simulink model "crazy_model_LQR"  (R2014b)
settings: Solver=ode4  StartTime=0.0  StopTime=1  FixedStep=0.01  RelTol=1e-3
values from neighbouring files (symbols this model uses):
  Engine_back = 1.3    [main.m]
  Engine_front = 1.3    [main.m]
  Engine_left = 1.3    [main.m]
  Engine_right = 1.3    [main.m]
  Klqr = [-0.0000   -0.5502   -0.0000   -0.0000   -0.0516   -0.0000    0.0000   -0.8559    0.6891    0.0000   -0.2911    0.2725 ... (first row only)    [C_code_Klqr.m]    (also in main.m = lqr(A,B,Qx,Qu))
  Kv = 14000*[1 0 0 0 ... (first row only)    [control_PWM.m]    (also in linearize_pwm.m = 14000; linearize_voltage.m = 14000; main.m)
settings Model: Creator=Abhiram  LastModifiedBy=Abhiram

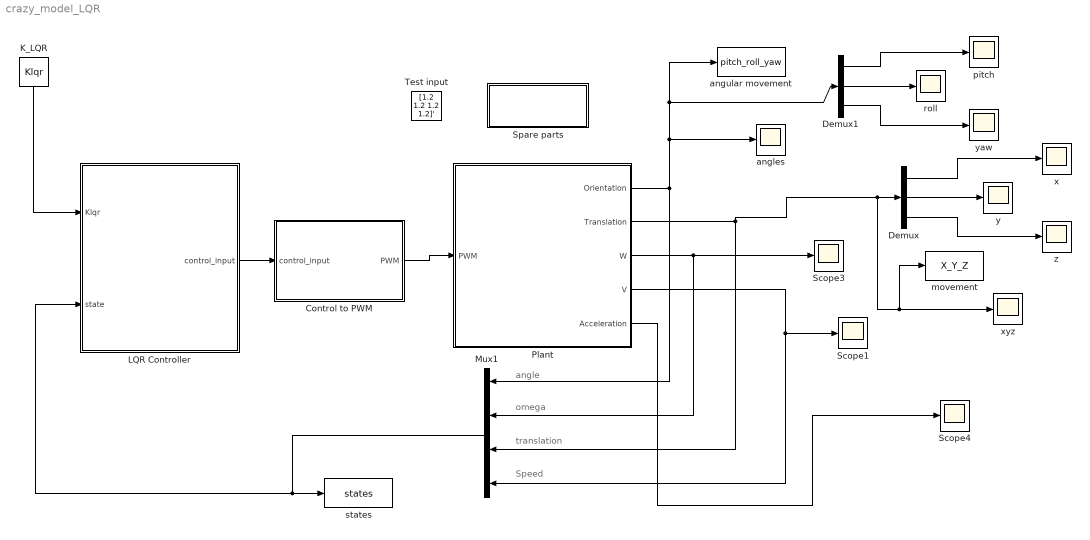
== system crazy_model_LQR ==
  note: Speed
  note: translation
  note: omega
  note: angle
  Control to PWM : MATLAB Function  TreatAsAtomicUnit=on
  Demux : Demux  Outputs=3
  Demux1 : Demux  Outputs=3
  K_LQR : Constant  Value=Klqr
  LQR Controller : MATLAB Function  TreatAsAtomicUnit=on
  Mux1 : Mux
  Plant : Subsystem
  Scope1 : Scope
  Scope3 : Scope
      settings: SaveName=ScopeData3
  Scope4 : Scope
      settings: SaveName=ScopeData4
  Spare parts : Subsystem
  Test input : Constant  Value=[1.2 1.2 1.2 1.2]'
  angles : Scope
      settings: SaveName=ScopeData10
  angular movement : ToWorkspace  VariableName=pitch_roll_yaw  SaveFormat=Structure With Time  SampleTime=-1
  movement : ToWorkspace  VariableName=X_Y_Z  SaveFormat=Structure With Time  SampleTime=-1
  pitch : Scope
  roll : Scope
      settings: TimeRange=10  YMin=0  YMax=25  SaveName=ScopeData7
  states : ToWorkspace  VariableName=states  SaveFormat=Structure With Time  SampleTime=-1
  x : Scope
      settings: SaveName=ScopeData2
  xyz : Scope
      settings: TimeRange=10  YMin=-20  YMax=120  SaveName=ScopeData9
  y : Scope
      settings: SaveName=ScopeData5
  yaw : Scope
      settings: SaveName=ScopeData8
  z : Scope
      settings: SaveName=ScopeData6
  wires:
  Plant/1(Orientation) -> angular movement/1, Demux1/1, angles/1, Mux1/1
  Plant/3(W) -> Mux1/2, Scope3/1
  Plant/4(V) -> Mux1/4, Scope1/1
  Plant/5(Acceleration) -> Scope4/1
  Plant/2(Translation) -> Demux/1, movement/1, xyz/1, Mux1/3
  Demux/1 -> x/1
  Demux/2 -> y/1
  Demux/3 -> z/1
  Demux1/1 -> pitch/1
  Demux1/2 -> roll/1
  Demux1/3 -> yaw/1
  Mux1/1 -> states/1, LQR Controller/2(state)
  Control to PWM/1(PWM) -> Plant/1(PWM)
  LQR Controller/1(control_input) -> Control to PWM/1(control_input)
  K_LQR/1 -> LQR Controller/1(Klqr)

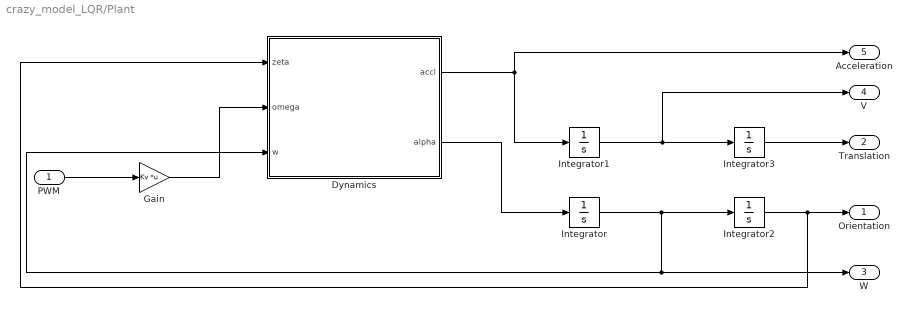
== system crazy_model_LQR/Plant ==
  PWM : Inport
  Dynamics : MATLAB Function  TreatAsAtomicUnit=on
  Gain : Gain  Gain=Kv  Multiplication=Matrix(K*u)
  Integrator{,1..3} (4 alike) : Integrator  InitialCondition=[0 0 0]'
  Orientation : Outport
  Translation : Outport  Port=2
  W : Outport  Port=3
  V : Outport  Port=4
  Acceleration : Outport  Port=5
  wires:
  Integrator/1 -> Integrator2/1, W/1, Dynamics/3(w)
  Integrator1/1 -> V/1, Integrator3/1
  Integrator2/1 -> Dynamics/1(zeta), Orientation/1
  Integrator3/1 -> Translation/1
  PWM/1 -> Gain/1
  Dynamics/2(alpha) -> Integrator/1
  Dynamics/1(accl) -> Integrator1/1, Acceleration/1
  Gain/1 -> Dynamics/2(omega)

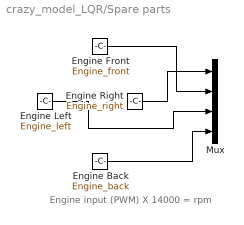
== system crazy_model_LQR/Spare parts ==
  note: Engine input (PWM) X 14000 = rpm
  Engine Back : Constant  Value=Engine_back
  Engine Front : Constant  Value=Engine_front
  Engine Left : Constant  Value=Engine_left
  Engine Right : Constant  Value=Engine_right
  Mux : Mux
  wires:
  Engine Right/1 -> Mux/1
  Engine Front/1 -> Mux/2
  Engine Left/1 -> Mux/3
  Engine Back/1 -> Mux/4

== matlab function crazy_model_LQR/Plant/Dynamics ==
  data: zeta input; omega input; accl output; alpha output; w input
function [accl, alpha] = fcn(zeta, omega, w)

    Ixx = 2.09*10^(-05);
    Iyy = 2.09*10^(-05);
    Izz = 3.81*10^(-05);
    I = diag([Ixx,Iyy,Izz]);                              % Inertia matrix - needs revision

    d = 0.046;
    m = 0.027;
    g = 9.8;

%%%%%%%%%%%%%%%%%%%%%%%%%%%%%%%%%%%%%%%%%%%%%%%%%%%%%%%%%%%%%%%%%%%%%%%%%%%
%3
    theta = zeta(1);         % pitch    
    phi = zeta(2);           % roll
    psi = zeta(3);           % yaw  
    
% %     omega_square = [omega(1)^2 omega(2)^2 omega(3)^2 omega(4)^2]';
% %     T_b = C*omega_square;    
% %     %     C = [Ct     Ct    Ct    Ct;
% %     %          0      d*Ct  0     -d*Ct;
% %     %         -d*Ct   0     d*Ct  0;
% %     %         -Cq     Cq   -Cq    Cq ]; % Plus config
    
    [T_b] = thrust(omega);              % non linear function for thrust
    
    F_e = T_b(1)*[-sin(theta); cos(theta)*sin(phi); cos(theta)*cos(phi)];
    
    Tau_e = [T_b(2) T_b(3) T_b(4)]';
    G = [0 0 m*g]';

    T_e = [F_e - G; Tau_e];

    I_a = [m*eye(3)    zeros(3,3);
           zeros(3,3)         I ];

    w_cross = cross(w,I*w);

    % Needs Revision
    A = I_a \ ( T_e - [0;0;0;w_cross] );
    
    accl = A(1:3);
    alpha = A(4:6);

end

== matlab function crazy_model_LQR/LQR Controller ==
  data: Klqr input; control_input output; state input
function control_input = fcn(Klqr, state)
% function control_input = fcn(Qu, Qx, A, B, constant, state)

control_input = -Klqr*(state);
%control_input = -Klqr*(state + A\constant);
end

== matlab function crazy_model_LQR/Control to PWM ==
  data: control_input input; PWM output
function PWM = fcn(control_input)
% Provides PWM signal for perticular control input

Ct = 1.0942e-07;
C1 = 0.25*(Ct)*9.8/1000;                                                    % grams to newton                           
Cq = 1*(10^(-9))*(60/(2*pi))^2;                                             % Cq in rpm
d = 0.046;

Kv =  14000*[1 0 0 0
             0 1 0 0
             0 0 1 0
             0 0 0 1]';

B = control_input;

A = [  C1   C1    C1    C1;
       0    d*C1  0    -d*C1;
      -d*C1 0     d*C1  0;
      -Cq   Cq   -Cq    Cq];

X = linsolve(A,B);

% w1 = sqrt(X(1));
% w2 = sqrt(X(2));
% w3 = sqrt(X(3));
% w4 = sqrt(X(4));

w1 = (X(1));
w2 = (X(2));
w3 = (X(3));
w4 = (X(4));

PWM = Kv\[w1; w2; w3; w4];

end
